simulink model "ik_sim"  (R2019b)
settings: Solver=VariableStepAuto  StartTime=0.0  StopTime=t_k  FixedStep=t_s  MaxStep=t_s  RelTol=1e-3
values from neighbouring files (symbols this model uses):
  d_r = [0.01 0.01 0.01 0.01 0.01 0.01]    [model.mat]
  Fi_b_z = in_rlb(12,1)    [fcn_s_rlb.m]    (also in fcn_s_rub.m = in_rub(12,1); model.mat = [0 2.09439510239 4.18879020479 1.0471975512 3.14159265359 5.)
  l_r = in_rlb(3,1)    [fcn_s_rlb.m]    (also in fcn_s_rub.m = in_rub(3,1); model.mat = [0.36 0.36 0.36 0.36 0.36 0.36])
  O_lb = in_rlb(4:9,1)    [fcn_s_rlb.m]    (also in model.mat = [0 0 0 0 0 0])
  w_lb = in_rlb(11,1)    [fcn_s_rlb.m]    (also in model.mat = 0.195)
  W_lb = 0.205    [model.mat]
  w_ub = in_rub(11,1)    [fcn_s_rub.m]    (also in model.mat = 0.195)
  W_ub = 0.205    [model.mat]
undefined symbols (not defined in the file or in its folder): amp, l_b, om, s_b, t_0, X, Y, Z
libraries: nesl_utility x145, sm_lib x111, dspindex x18
(part 1 of 7)
settings Model: Creator=Vojta  LastModifiedBy=Tom

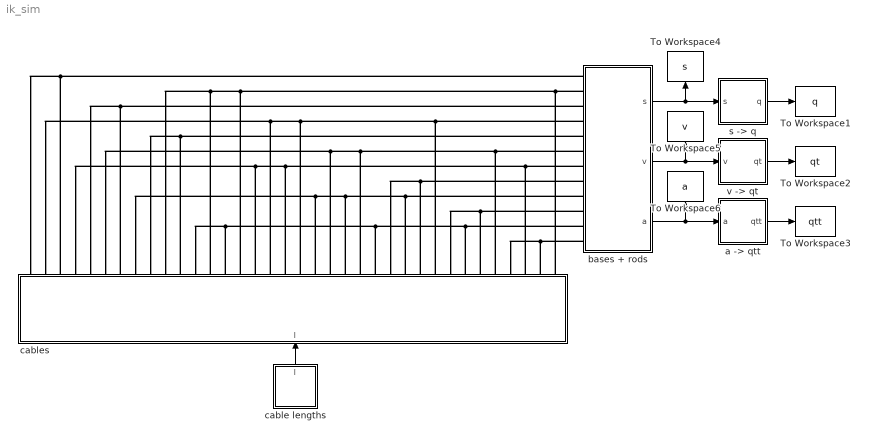
== system ik_sim ==
  To Workspace1 : ToWorkspace  VariableName=q  SampleTime=-1
  To Workspace2 : ToWorkspace  VariableName=qt  SampleTime=-1
  To Workspace3 : ToWorkspace  VariableName=qtt  SampleTime=-1
  To Workspace4 : ToWorkspace  VariableName=s  SampleTime=-1
  To Workspace5 : ToWorkspace  VariableName=v  SampleTime=-1
  To Workspace6 : ToWorkspace  VariableName=a  SampleTime=-1
  "a -> qtt" : MATLAB Function  TreatAsAtomicUnit=on
  bases + rods : Subsystem
  cable lengths : Subsystem
  cables : Subsystem
  "s -> q" : MATLAB Function  TreatAsAtomicUnit=on
  "v -> qt" : MATLAB Function  TreatAsAtomicUnit=on
  wires:
  bases + rods/1(s) -> "s -> q"/1(s), To Workspace4/1
  bases + rods/2(v) -> "v -> qt"/1(v), To Workspace5/1
  bases + rods/3(a) -> "a -> qtt"/1(a), To Workspace6/1
  "a -> qtt"/1(qtt) -> To Workspace3/1
  "v -> qt"/1(qt) -> To Workspace2/1
  "s -> q"/1(q) -> To Workspace1/1
  cable lengths/1(l) -> cables/1(l)
  connections:
  bases + rods/LConn1 -- cables/RConn3 -- cables/RConn1
  bases + rods/LConn2 -- cables/RConn36 -- cables/RConn15 -- cables/RConn10 -- cables/RConn13
  bases + rods/LConn3 -- cables/RConn7 -- cables/RConn5
  bases + rods/LConn4 -- cables/RConn28 -- cables/RConn19 -- cables/RConn17 -- cables/RConn2
  bases + rods/LConn5 -- cables/RConn11 -- cables/RConn9
  bases + rods/LConn6 -- cables/RConn32 -- cables/RConn23 -- cables/RConn21 -- cables/RConn6
  bases + rods/LConn7 -- cables/RConn34 -- cables/RConn18 -- cables/RConn16 -- cables/RConn4
  bases + rods/LConn8 -- cables/RConn27 -- cables/RConn25
  bases + rods/LConn9 -- cables/RConn26 -- cables/RConn22 -- cables/RConn20 -- cables/RConn8
  bases + rods/LConn10 -- cables/RConn31 -- cables/RConn29
  bases + rods/LConn11 -- cables/RConn30 -- cables/RConn24 -- cables/RConn14 -- cables/RConn12
  bases + rods/LConn12 -- cables/RConn35 -- cables/RConn33

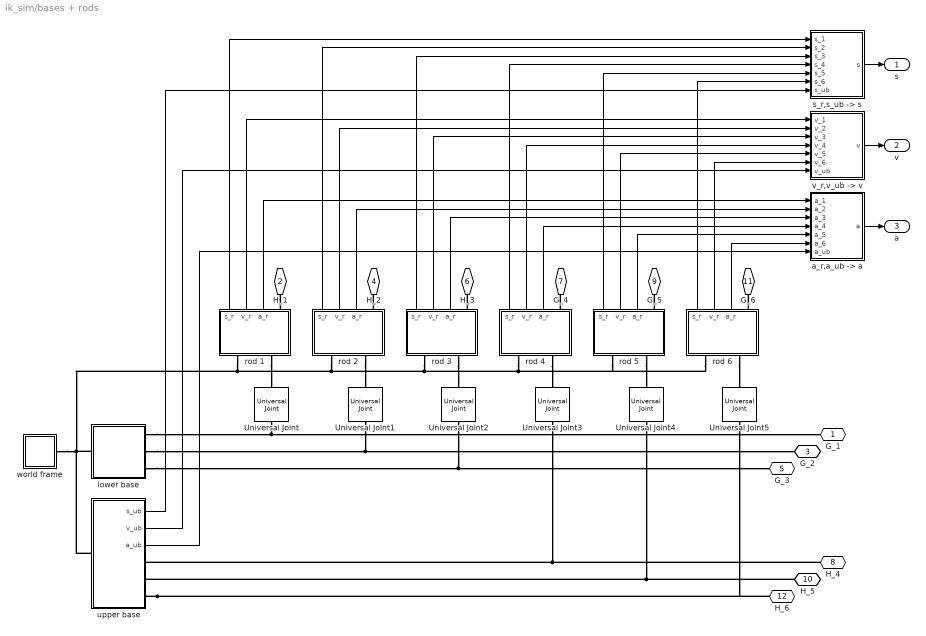
== system ik_sim/bases + rods ==
  Universal Joint{,1..5} (6 alike) : sm_lib/Joints/Universal Joint  JointMode=Normal  SenseConstraintForce=off  SenseConstraintForceX=off  SenseConstraintForceY=off  SenseConstraintForceZ=off  SenseConstraintTorque=off  SenseConstraintTorqueX=off  SenseConstraintTorqueY=off  SenseConstraintTorqueZ=off  SenseTotalForce=off  SenseTotalForceX=off  SenseTotalForceY=off  SenseTotalForceZ=off  SenseTotalTorque=off  SenseTotalTorqueX=off  SenseTotalTorqueY=off  SenseTotalTorqueZ=off  CompositeWrenchDir=FollowerOnBase  CompositeWrenchFrame=BaseFrame  RxEquilibriumPosition=0  RxEquilibriumPositionUnits=deg  RxSpringStiffness=0  RxSpringStiffnessUnits=N*m/deg  RxDampingCoefficient=0  RxDampingCoefficientUnits=N*m/(deg/s)  RxTorqueActuationMode=NoTorque  RxMotionActuationMode=ComputedMotion  RxSensePosition=off  RxSenseVelocity=off  RxSenseAcceleration=off  RxSenseTorqueForce=off  RxSenseLowerLimitTorqueForce=off  RxSenseUpperLimitTorqueForce=off  RxLowerLimitSpecify=off  RxLowerLimitBound=-90  RxLowerLimitBoundUnits=deg  RxLowerLimitStiffness=1e4  RxLowerLimitStiffnessUnits=N*m/deg  RxLowerLimitDamping=10  RxLowerLimitDampingUnits=N*m/(deg/s)  RxLowerLimitTransitionRegionWidth=0.1  RxLowerLimitTransitionRegionWidthUnits=deg  RxUpperLimitSpecify=off  RxUpperLimitBound=90  RxUpperLimitBoundUnits=deg  RxUpperLimitStiffness=1e4  RxUpperLimitStiffnessUnits=N*m/deg  RxUpperLimitDamping=10  RxUpperLimitDampingUnits=N*m/(deg/s)  RxUpperLimitTransitionRegionWidth=0.1  RxUpperLimitTransitionRegionWidthUnits=deg  RxPositionTargetSpecify=off  RxPositionTargetPriority=High  RxPositionTargetValue=0  RxPositionTargetValueUnits=deg  RxVelocityTargetSpecify=off  RxVelocityTargetPriority=High  RxVelocityTargetValue=0  RxVelocityTargetValueUnits=deg/s  RyEquilibriumPosition=0  RyEquilibriumPositionUnits=deg  RySpringStiffness=0  RySpringStiffnessUnits=N*m/deg  RyDampingCoefficient=0  RyDampingCoefficientUnits=N*m/(deg/s)  RyTorqueActuationMode=NoTorque  RyMotionActuationMode=ComputedMotion  RySensePosition=off  RySenseVelocity=off  RySenseAcceleration=off  RySenseTorqueForce=off  RySenseLowerLimitTorqueForce=off  RySenseUpperLimitTorqueForce=off  RyLowerLimitSpecify=off  RyLowerLimitBound=-90  RyLowerLimitBoundUnits=deg  RyLowerLimitStiffness=1e4  RyLowerLimitStiffnessUnits=N*m/deg  RyLowerLimitDamping=10  RyLowerLimitDampingUnits=N*m/(deg/s)  RyLowerLimitTransitionRegionWidth=0.1  RyLowerLimitTransitionRegionWidthUnits=deg  RyUpperLimitSpecify=off  RyUpperLimitBound=90  RyUpperLimitBoundUnits=deg  RyUpperLimitStiffness=1e4  RyUpperLimitStiffnessUnits=N*m/deg  RyUpperLimitDamping=10  RyUpperLimitDampingUnits=N*m/(deg/s)  RyUpperLimitTransitionRegionWidth=0.1  RyUpperLimitTransitionRegionWidthUnits=deg  RyPositionTargetSpecify=off  RyPositionTargetPriority=High  RyPositionTargetValue=0  RyPositionTargetValueUnits=deg  RyVelocityTargetSpecify=off  RyVelocityTargetPriority=High  RyVelocityTargetValue=0  RyVelocityTargetValueUnits=deg/s
      settings: SourceProductName=Simscape Multibody
  "a_r,a_ub -> a" : MATLAB Function  TreatAsAtomicUnit=on
  lower base : Subsystem
  rod 1 : Subsystem  mask{r=1}
  rod 2 : Subsystem  mask{r=2}
  rod 3 : Subsystem  mask{r=3}
  rod 4 : Subsystem  mask{r=4}
  rod 5 : Subsystem  mask{r=5}
  rod 6 : Subsystem  mask{r=6}
  "s_r,s_ub -> s" : MATLAB Function  TreatAsAtomicUnit=on
  upper base : Subsystem
  "v_r,v_ub -> v" : MATLAB Function  TreatAsAtomicUnit=on
  world frame : Subsystem
  G_1 : PMIOPort  Side=Left
  H_1 : PMIOPort  Port=2  Side=Left
  G_2 : PMIOPort  Port=3  Side=Left
  H_2 : PMIOPort  Port=4  Side=Left
  G_3 : PMIOPort  Port=5  Side=Left
  H_3 : PMIOPort  Port=6  Side=Left
  G_4 : PMIOPort  Port=7  Side=Left
  H_4 : PMIOPort  Port=8  Side=Left
  G_5 : PMIOPort  Port=9  Side=Left
  H_5 : PMIOPort  Port=10  Side=Left
  G_6 : PMIOPort  Port=11  Side=Left
  H_6 : PMIOPort  Port=12  Side=Left
  s : Outport
  v : Outport  Port=2
  a : Outport  Port=3
  wires:
  "a_r,a_ub -> a"/1(a) -> a/1
  rod 1/1(s_r) -> "s_r,s_ub -> s"/1(s_1)
  rod 2/1(s_r) -> "s_r,s_ub -> s"/2(s_2)
  rod 3/1(s_r) -> "s_r,s_ub -> s"/3(s_3)
  rod 4/1(s_r) -> "s_r,s_ub -> s"/4(s_4)
  rod 5/1(s_r) -> "s_r,s_ub -> s"/5(s_5)
  rod 6/1(s_r) -> "s_r,s_ub -> s"/6(s_6)
  upper base/1(s_ub) -> "s_r,s_ub -> s"/7(s_ub)
  upper base/2(v_ub) -> "v_r,v_ub -> v"/7(v_ub)
  upper base/3(a_ub) -> "a_r,a_ub -> a"/7(a_ub)
  rod 1/2(v_r) -> "v_r,v_ub -> v"/1(v_1)
  rod 2/2(v_r) -> "v_r,v_ub -> v"/2(v_2)
  rod 3/2(v_r) -> "v_r,v_ub -> v"/3(v_3)
  rod 4/2(v_r) -> "v_r,v_ub -> v"/4(v_4)
  rod 5/2(v_r) -> "v_r,v_ub -> v"/5(v_5)
  rod 6/2(v_r) -> "v_r,v_ub -> v"/6(v_6)
  rod 1/3(a_r) -> "a_r,a_ub -> a"/1(a_1)
  rod 2/3(a_r) -> "a_r,a_ub -> a"/2(a_2)
  rod 3/3(a_r) -> "a_r,a_ub -> a"/3(a_3)
  rod 4/3(a_r) -> "a_r,a_ub -> a"/4(a_4)
  rod 5/3(a_r) -> "a_r,a_ub -> a"/5(a_5)
  rod 6/3(a_r) -> "a_r,a_ub -> a"/6(a_6)
  "v_r,v_ub -> v"/1(v) -> v/1
  "s_r,s_ub -> s"/1(s) -> s/1
  connections:
  Universal Joint2/LConn1 -- G_3/RConn1 -- lower base/RConn3
  Universal Joint1/LConn1 -- G_2/RConn1 -- lower base/RConn2
  H_4/RConn1 -- Universal Joint3/LConn1 -- upper base/RConn1
  Universal Joint/LConn1 -- G_1/RConn1 -- lower base/RConn1
  rod 1/LConn1 -- rod 2/LConn1 -- rod 3/LConn1 -- rod 4/LConn1 -- rod 6/LConn1 -- rod 5/LConn1 -- world frame/RConn1 -- upper base/LConn1 -- lower base/LConn1
  upper base/RConn3 -- H_6/RConn1 -- Universal Joint5/LConn1
  H_5/RConn1 -- Universal Joint4/LConn1 -- upper base/RConn2
  rod 1/RConn1 -- H_1/RConn1
  rod 1/LConn2 -- Universal Joint/RConn1
  rod 2/LConn2 -- Universal Joint1/RConn1
  rod 3/LConn2 -- Universal Joint2/RConn1
  rod 2/RConn1 -- H_2/RConn1
  rod 3/RConn1 -- H_3/RConn1
  rod 4/LConn2 -- Universal Joint3/RConn1
  rod 4/RConn1 -- G_4/RConn1
  rod 5/LConn2 -- Universal Joint4/RConn1
  rod 6/LConn2 -- Universal Joint5/RConn1
  rod 5/RConn1 -- G_5/RConn1
  rod 6/RConn1 -- G_6/RConn1

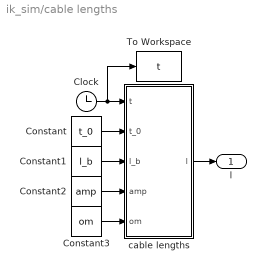
== system ik_sim/cable lengths ==
  Clock : Clock
  Constant : Constant  Value=t_0
  Constant1 : Constant  Value=l_b
  Constant2 : Constant  Value=amp
  Constant3 : Constant  Value=om
  To Workspace : ToWorkspace  VariableName=t  SampleTime=-1
  cable lengths : MATLAB Function  TreatAsAtomicUnit=on
  l : Outport
  wires:
  Constant/1 -> cable lengths/2(t_0)
  Constant1/1 -> cable lengths/3(l_b)
  Constant2/1 -> cable lengths/4(amp)
  Constant3/1 -> cable lengths/5(om)
  Clock/1 -> To Workspace/1, cable lengths/1(t)
  cable lengths/1(l) -> l/1

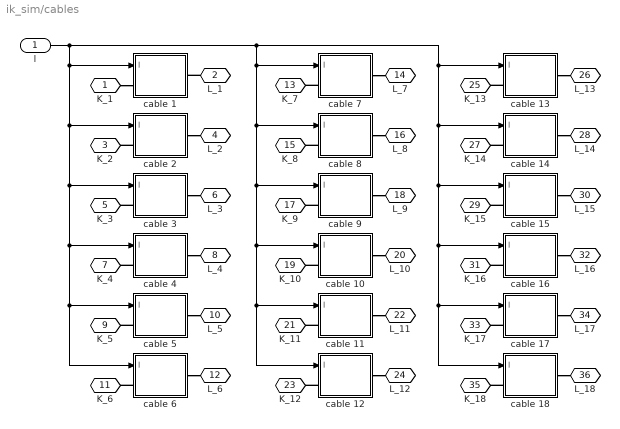
== system ik_sim/cables ==
  l : Inport
  cable 1 : Subsystem  mask{c=1}
  cable 10 : Subsystem  mask{c=10}
  cable 11 : Subsystem  mask{c=11}
  cable 12 : Subsystem  mask{c=12}
  cable 13 : Subsystem  mask{c=13}
  cable 14 : Subsystem  mask{c=14}
  cable 15 : Subsystem  mask{c=15}
  cable 16 : Subsystem  mask{c=16}
  cable 17 : Subsystem  mask{c=17}
  cable 18 : Subsystem  mask{c=18}
  cable 2 : Subsystem  mask{c=2}
  cable 3 : Subsystem  mask{c=3}
  cable 4 : Subsystem  mask{c=4}
  cable 5 : Subsystem  mask{c=5}
  cable 6 : Subsystem  mask{c=6}
  cable 7 : Subsystem  mask{c=7}
  cable 8 : Subsystem  mask{c=8}
  cable 9 : Subsystem  mask{c=9}
  K_1 : PMIOPort  Side=Right
  L_1 : PMIOPort  Port=2  Side=Right
  K_2 : PMIOPort  Port=3  Side=Right
  L_2 : PMIOPort  Port=4  Side=Right
  K_3 : PMIOPort  Port=5  Side=Right
  L_3 : PMIOPort  Port=6  Side=Right
  K_4 : PMIOPort  Port=7  Side=Right
  L_4 : PMIOPort  Port=8  Side=Right
  K_5 : PMIOPort  Port=9  Side=Right
  L_5 : PMIOPort  Port=10  Side=Right
  K_6 : PMIOPort  Port=11  Side=Right
  L_6 : PMIOPort  Port=12  Side=Right
  K_7 : PMIOPort  Port=13  Side=Right
  L_7 : PMIOPort  Port=14  Side=Right
  K_8 : PMIOPort  Port=15  Side=Right
  L_8 : PMIOPort  Port=16  Side=Right
  K_9 : PMIOPort  Port=17  Side=Right
  L_9 : PMIOPort  Port=18  Side=Right
  K_10 : PMIOPort  Port=19  Side=Right
  L_10 : PMIOPort  Port=20  Side=Right
  K_11 : PMIOPort  Port=21  Side=Right
  L_11 : PMIOPort  Port=22  Side=Right
  K_12 : PMIOPort  Port=23  Side=Right
  L_12 : PMIOPort  Port=24  Side=Right
  K_13 : PMIOPort  Port=25  Side=Right
  L_13 : PMIOPort  Port=26  Side=Right
  K_14 : PMIOPort  Port=27  Side=Right
  L_14 : PMIOPort  Port=28  Side=Right
  K_15 : PMIOPort  Port=29  Side=Right
  L_15 : PMIOPort  Port=30  Side=Right
  K_16 : PMIOPort  Port=31  Side=Right
  L_16 : PMIOPort  Port=32  Side=Right
  K_17 : PMIOPort  Port=33  Side=Right
  L_17 : PMIOPort  Port=34  Side=Right
  K_18 : PMIOPort  Port=35  Side=Right
  L_18 : PMIOPort  Port=36  Side=Right
  wires:
  l/1 -> cable 1/1(l), cable 2/1(l), cable 3/1(l), cable 4/1(l), cable 5/1(l), cable 6/1(l), cable 7/1(l), cable 8/1(l), cable 9/1(l), cable 10/1(l), cable 12/1(l), cable 11/1(l), cable 13/1(l), cable 14/1(l), cable 15/1(l), cable 16/1(l), cable 18/1(l), cable 17/1(l)
  connections:
  L_1/RConn1 -- cable 1/RConn1
  K_1/RConn1 -- cable 1/LConn1
  cable 2/LConn1 -- K_2/RConn1
  cable 2/RConn1 -- L_2/RConn1
  cable 3/LConn1 -- K_3/RConn1
  cable 4/LConn1 -- K_4/RConn1
  cable 5/LConn1 -- K_5/RConn1
  cable 6/LConn1 -- K_6/RConn1
  cable 9/RConn1 -- L_9/RConn1
  cable 9/LConn1 -- K_9/RConn1
  cable 7/RConn1 -- L_7/RConn1
  cable 7/LConn1 -- K_7/RConn1
  cable 8/RConn1 -- L_8/RConn1
  cable 8/LConn1 -- K_8/RConn1
  cable 11/LConn1 -- K_11/RConn1
  cable 10/RConn1 -- L_10/RConn1
  cable 11/RConn1 -- L_11/RConn1
  cable 12/RConn1 -- L_12/RConn1
  cable 12/LConn1 -- K_12/RConn1
  cable 10/LConn1 -- K_10/RConn1
  cable 13/LConn1 -- K_13/RConn1
  cable 14/RConn1 -- L_14/RConn1
  cable 13/RConn1 -- L_13/RConn1
  cable 15/RConn1 -- L_15/RConn1
  cable 14/LConn1 -- K_14/RConn1
  cable 15/LConn1 -- K_15/RConn1
  cable 17/RConn1 -- L_17/RConn1
  cable 18/LConn1 -- K_18/RConn1
  cable 16/RConn1 -- L_16/RConn1
  cable 17/LConn1 -- K_17/RConn1
  cable 18/RConn1 -- L_18/RConn1
  cable 16/LConn1 -- K_16/RConn1
  cable 3/RConn1 -- L_3/RConn1
  cable 4/RConn1 -- L_4/RConn1
  cable 5/RConn1 -- L_5/RConn1
  cable 6/RConn1 -- L_6/RConn1

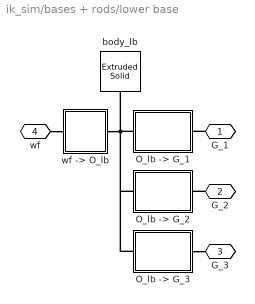
== system ik_sim/bases + rods/lower base ==
  "O_lb -> G_1" : Subsystem
  "O_lb -> G_2" : Subsystem
  "O_lb -> G_3" : Subsystem
  body_lb : sm_lib/Body Elements/Extruded Solid  GraphicAmbientColor=[0.15 0.15 0.15 1.0]  BasedOnType=Density  CenterOfMass=[0 0 0]  CenterOfMassUnits=m  GraphicDiffuseColor=[0.5,0.5,0.5]  ExtrusionCrossSection=[1 1; -1 1; -1 -1; 1 -1]  ExtrusionCrossSectionUnits=m  Density=Ro_lb  DensityUnits=kg/m^3  DoExposeReferenceFrame=on  GraphicEmissiveColor=[0.0 0.0 0.0 1.0]  ExportEntireGeometry=off  ExtrusionLength=t_lb  ExtrusionLengthUnits=m  ExtrusionType=Regular  SerializedFrames=<Frames/>  MarkerShape=Sphere  MarkerSize=10  GraphicType=FromGeometry  InertiaType=CalculateFromGeometry  Mass=1  MassUnits=kg  MomentsOfInertia=[1 1 1]  MomentsOfInertiaUnits=kg*m^2  PolygonNumSides=6  GraphicOpacity=1  PolygonOuterRadius=(W_lb/2)/cosd(30)  PolygonOuterRadiusUnits=m  ProductsOfInertia=[0 0 0]  ProductsOfInertiaUnits=kg*m^2  GraphicShininess=75  GraphicSpecularColor=[0.5 0.5 0.5 1.0]  GraphicVisPropType=SimpleVisualProperties
      settings: SourceProductName=Simscape Multibody
  "wf -> O_lb" : Subsystem
  G_1 : PMIOPort  Side=Right
  G_2 : PMIOPort  Port=2  Side=Right
  G_3 : PMIOPort  Port=3  Side=Right
  wf : PMIOPort  Port=4  Side=Left
  connections:
  wf/RConn1 -- "wf -> O_lb"/LConn1
  "wf -> O_lb"/RConn1 -- "O_lb -> G_3"/LConn1 -- "O_lb -> G_2"/LConn1 -- body_lb/RConn1 -- "O_lb -> G_1"/LConn1
  G_1/RConn1 -- "O_lb -> G_1"/RConn1
  G_2/RConn1 -- "O_lb -> G_2"/RConn1
  "O_lb -> G_3"/RConn1 -- G_3/RConn1

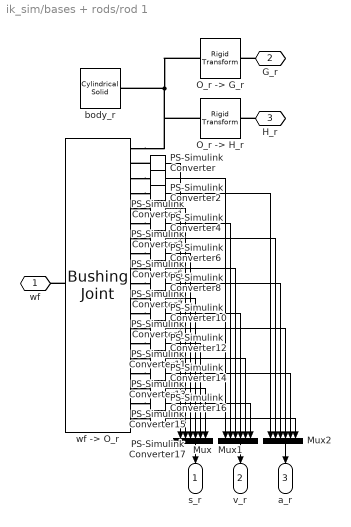
== system ik_sim/bases + rods/rod 1 ==
  Mux : Mux  Inputs=6
  Mux1 : Mux  Inputs=6
  Mux2 : Mux  Inputs=6
  "O_r -> G_r" : sm_lib/Frames and Transforms/Rigid Transform  TranslationMethod=StandardAxis  TranslationStandardOffset=l_r(r)/2  TranslationLengthUnit=m  TranslationStandardAxis=-Z  TranslationCartesianOffset=[0 0 0]  TranslationROffset=0  TranslationROffsetUnits=m  TranslationZOffset=0  TranslationZOffsetUnits=m  TranslationThetaOffset=0  TranslationThetaOffsetUnits=deg  RotationMethod=None  RotationAngleUnits=deg  RotationStandardAxis=+Z  RotationAngle=0.0  RotationArbitraryAxis=[0 0 1]  FollAlignAxisA=+X  BaseAlignAxisA=+Y  FollAlignAxisB=+Y  BaseAlignAxisB=+Z  RotationSequenceAxes=FollowerAxes  RotationSequence=XYX  RotationSequenceAngles=[0 0 0]  RotationSequenceAnglesUnits=deg  RotationMatrix=[1 0 0; 0 1 0; 0 0 1]
  "O_r -> H_r" : sm_lib/Frames and Transforms/Rigid Transform  TranslationMethod=StandardAxis  TranslationStandardOffset=l_r(r)/2  TranslationLengthUnit=m  TranslationStandardAxis=+Z  TranslationCartesianOffset=[0 0 0]  TranslationROffset=0  TranslationROffsetUnits=m  TranslationZOffset=0  TranslationZOffsetUnits=m  TranslationThetaOffset=0  TranslationThetaOffsetUnits=deg  RotationMethod=None  RotationAngleUnits=deg  RotationStandardAxis=+Z  RotationAngle=0.0  RotationArbitraryAxis=[0 0 1]  FollAlignAxisA=+X  BaseAlignAxisA=+Y  FollAlignAxisB=+Y  BaseAlignAxisB=+Z  RotationSequenceAxes=FollowerAxes  RotationSequence=XYX  RotationSequenceAngles=[0 0 0]  RotationSequenceAnglesUnits=deg  RotationMatrix=[1 0 0; 0 1 0; 0 0 1]
  PS-Simulink Converter{,1..17} (18 alike) : nesl_utility/PS-Simulink Converter  PhysicalDomain=network_engine_domain  SubClassName=ps_output  LeftPortType=input  RightPortType=output  PseudoPeriodic=off  Frequencies=[]  Unit=inherit  AffineConversion=off
  body_r : sm_lib/Body Elements/Cylindrical Solid  GraphicAmbientColor=[0.15 0.15 0.15 1.0]  BasedOnType=Density  CenterOfMass=[0 0 0]  CenterOfMassUnits=m  GraphicDiffuseColor=[0.5,0.5,0.5]  CylinderLength=l_r(r)  CylinderLengthUnits=m  CylinderRadius=d_r(r)/2  CylinderRadiusUnits=m  Density=Ro_r  DensityUnits=kg/m^3  DoExposeReferenceFrame=on  GraphicEmissiveColor=[0.0 0.0 0.0 1.0]  ExportEntireGeometry=off  SerializedFrames=<Frames/>  MarkerShape=Sphere  MarkerSize=10  GraphicType=FromGeometry  InertiaType=CalculateFromGeometry  Mass=1  MassUnits=kg  MomentsOfInertia=[1 1 1]  MomentsOfInertiaUnits=kg*m^2  GraphicOpacity=1  ProductsOfInertia=[0 0 0]  ProductsOfInertiaUnits=kg*m^2  GraphicShininess=75  GraphicSpecularColor=[0.5 0.5 0.5 1.0]  GraphicVisPropType=SimpleVisualProperties
  "wf -> O_r" : sm_lib/Joints/Bushing Joint  JointMode=Normal  SenseConstraintForce=off  SenseConstraintForceX=off  SenseConstraintForceY=off  SenseConstraintForceZ=off  SenseConstraintTorque=off  SenseConstraintTorqueX=off  SenseConstraintTorqueY=off  SenseConstraintTorqueZ=off  SenseTotalForce=off  SenseTotalForceX=off  SenseTotalForceY=off  SenseTotalForceZ=off  SenseTotalTorque=off  SenseTotalTorqueX=off  SenseTotalTorqueY=off  SenseTotalTorqueZ=off  CompositeWrenchDir=FollowerOnBase  CompositeWrenchFrame=BaseFrame  PxEquilibriumPosition=0  PxEquilibriumPositionUnits=m  PxSpringStiffness=0  PxSpringStiffnessUnits=N/m  PxDampingCoefficient=0  PxDampingCoefficientUnits=N/(m/s)  PxTorqueActuationMode=NoTorque  PxMotionActuationMode=ComputedMotion  PxSensePosition=on  PxSenseVelocity=on  PxSenseAcceleration=on  PxSenseTorqueForce=off  PxSenseLowerLimitTorqueForce=off  PxSenseUpperLimitTorqueForce=off  PxLowerLimitSpecify=off  PxLowerLimitBound=-1  PxLowerLimitBoundUnits=m  PxLowerLimitStiffness=1e6  PxLowerLimitStiffnessUnits=N/m  PxLowerLimitDamping=1e3  PxLowerLimitDampingUnits=N/(m/s)  PxLowerLimitTransitionRegionWidth=1e-4  PxLowerLimitTransitionRegionWidthUnits=m  PxUpperLimitSpecify=off  PxUpperLimitBound=1  PxUpperLimitBoundUnits=m  PxUpperLimitStiffness=1e6  PxUpperLimitStiffnessUnits=N/m  PxUpperLimitDamping=1e3  PxUpperLimitDampingUnits=N/(m/s)  PxUpperLimitTransitionRegionWidth=1e-4  PxUpperLimitTransitionRegionWidthUnits=m  PxPositionTargetSpecify=on  PxPositionTargetPriority=Low  PxPositionTargetValue=s_b(1,r)  PxPositionTargetValueUnits=m  PxVelocityTargetSpecify=off  PxVelocityTargetPriority=High  PxVelocityTargetValue=0  PxVelocityTargetValueUnits=m/s  PyEquilibriumPosition=0  PyEquilibriumPositionUnits=m  PySpringStiffness=0  PySpringStiffnessUnits=N/m  PyDampingCoefficient=0  PyDampingCoefficientUnits=N/(m/s)  PyTorqueActuationMode=NoTorque  PyMotionActuationMode=ComputedMotion  PySensePosition=on  PySenseVelocity=on  PySenseAcceleration=on  PySenseTorqueForce=off  PySenseLowerLimitTorqueForce=off  PySenseUpperLimitTorqueForce=off  PyLowerLimitSpecify=off  PyLowerLimitBound=-1  PyLowerLimitBoundUnits=m  PyLowerLimitStiffness=1e6  PyLowerLimitStiffnessUnits=N/m  PyLowerLimitDamping=1e3  PyLowerLimitDampingUnits=N/(m/s)  PyLowerLimitTransitionRegionWidth=1e-4  PyLowerLimitTransitionRegionWidthUnits=m  PyUpperLimitSpecify=off  PyUpperLimitBound=1  PyUpperLimitBoundUnits=m  PyUpperLimitStiffness=1e6  PyUpperLimitStiffnessUnits=N/m  PyUpperLimitDamping=1e3  PyUpperLimitDampingUnits=N/(m/s)  PyUpperLimitTransitionRegionWidth=1e-4  PyUpperLimitTransitionRegionWidthUnits=m  PyPositionTargetSpecify=on  PyPositionTargetPriority=Low  PyPositionTargetValue=s_b(2,r)  PyPositionTargetValueUnits=m  PyVelocityTargetSpecify=off  PyVelocityTargetPriority=High  PyVelocityTargetValue=0  PyVelocityTargetValueUnits=m/s  PzEquilibriumPosition=0  PzEquilibriumPositionUnits=m  PzSpringStiffness=0  PzSpringStiffnessUnits=N/m  PzDampingCoefficient=0  PzDampingCoefficientUnits=N/(m/s)  PzTorqueActuationMode=NoTorque  PzMotionActuationMode=ComputedMotion  PzSensePosition=on  PzSenseVelocity=on  PzSenseAcceleration=on  PzSenseTorqueForce=off  PzSenseLowerLimitTorqueForce=off  PzSenseUpperLimitTorqueForce=off  PzLowerLimitSpecify=off  PzLowerLimitBound=-1  PzLowerLimitBoundUnits=m  PzLowerLimitStiffness=1e6  PzLowerLimitStiffnessUnits=N/m  PzLowerLimitDamping=1e3  PzLowerLimitDampingUnits=N/(m/s)  PzLowerLimitTransitionRegionWidth=1e-4  PzLowerLimitTransitionRegionWidthUnits=m  PzUpperLimitSpecify=off  PzUpperLimitBound=1  PzUpperLimitBoundUnits=m  PzUpperLimitStiffness=1e6  PzUpperLimitStiffnessUnits=N/m  PzUpperLimitDamping=1e3  PzUpperLimitDampingUnits=N/(m/s)  PzUpperLimitTransitionRegionWidth=1e-4  PzUpperLimitTransitionRegionWidthUnits=m  PzPositionTargetSpecify=on  PzPositionTargetPriority=Low  PzPositionTargetValue=s_b(3,r)  PzPositionTargetValueUnits=m  PzVelocityTargetSpecify=off  PzVelocityTargetPriority=High  PzVelocityTargetValue=0  PzVelocityTargetValueUnits=m/s  RxEquilibriumPosition=0  RxEquilibriumPositionUnits=deg  RxSpringStiffness=0  RxSpringStiffnessUnits=N*m/deg  RxDampingCoefficient=0  RxDampingCoefficientUnits=N*m/(deg/s)  RxTorqueActuationMode=NoTorque  RxMotionActuationMode=ComputedMotion  RxSensePosition=on  RxSenseVelocity=on  RxSenseAcceleration=on  RxSenseTorqueForce=off  RxSenseLowerLimitTorqueForce=off  RxSenseUpperLimitTorqueForce=off  RxLowerLimitSpecify=off  RxLowerLimitBound=-90  RxLowerLimitBoundUnits=deg  RxLowerLimitStiffness=1e4  RxLowerLimitStiffnessUnits=N*m/deg  RxLowerLimitDamping=10  RxLowerLimitDampingUnits=N*m/(deg/s)  RxLowerLimitTransitionRegionWidth=0.1  RxLowerLimitTransitionRegionWidthUnits=deg  RxUpperLimitSpecify=off  RxUpperLimitBound=90  RxUpperLimitBoundUnits=deg  RxUpperLimitStiffness=1e4  RxUpperLimitStiffnessUnits=N*m/deg  RxUpperLimitDamping=10  RxUpperLimitDampingUnits=N*m/(deg/s)  RxUpperLimitTransitionRegionWidth=0.1  RxUpperLimitTransitionRegionWidthUnits=deg  RxPositionTargetSpecify=on  RxPositionTargetPriority=Low  RxPositionTargetValue=s_b(4,r)  RxPositionTargetValueUnits=rad  RxVelocityTargetSpecify=off  RxVelocityTargetPriority=High  RxVelocityTargetValue=0  RxVelocityTargetValueUnits=rad/s  RyEquilibriumPosition=0  RyEquilibriumPositionUnits=deg  RySpringStiffness=0  RySpringStiffnessUnits=N*m/deg  RyDampingCoefficient=0  RyDampingCoefficientUnits=N*m/(deg/s)  RyTorqueActuationMode=NoTorque  RyMotionActuationMode=ComputedMotion  RySensePosition=on  RySenseVelocity=on  RySenseAcceleration=on  RySenseTorqueForce=off  RySenseLowerLimitTorqueForce=off  RySenseUpperLimitTorqueForce=off  RyLowerLimitSpecify=off  RyLowerLimitBound=-90  RyLowerLimitBoundUnits=deg  RyLowerLimitStiffness=1e4  RyLowerLimitStiffnessUnits=N*m/deg  RyLowerLimitDamping=10  RyLowerLimitDampingUnits=N*m/(deg/s)  RyLowerLimitTransitionRegionWidth=0.1  RyLowerLimitTransitionRegionWidthUnits=deg  RyUpperLimitSpecify=off  RyUpperLimitBound=90  RyUpperLimitBoundUnits=deg  RyUpperLimitStiffness=1e4  RyUpperLimitStiffnessUnits=N*m/deg  RyUpperLimitDamping=10  RyUpperLimitDampingUnits=N*m/(deg/s)  RyUpperLimitTransitionRegionWidth=0.1  RyUpperLimitTransitionRegionWidthUnits=deg  RyPositionTargetSpecify=on  RyPositionTargetPriority=Low  RyPositionTargetValue=s_b(5,r)  RyPositionTargetValueUnits=rad  RyVelocityTargetSpecify=off  RyVelocityTargetPriority=High  RyVelocityTargetValue=0  RyVelocityTargetValueUnits=rad/s  RzEquilibriumPosition=0  RzEquilibriumPositionUnits=deg  RzSpringStiffness=0  RzSpringStiffnessUnits=N*m/deg  RzDampingCoefficient=0  RzDampingCoefficientUnits=N*m/(deg/s)  RzTorqueActuationMode=NoTorque  RzMotionActuationMode=ComputedMotion  RzSensePosition=on  RzSenseVelocity=on  RzSenseAcceleration=on  RzSenseTorqueForce=off  RzSenseLowerLimitTorqueForce=off  RzSenseUpperLimitTorqueForce=off  RzLowerLimitSpecify=off  RzLowerLimitBound=-90  RzLowerLimitBoundUnits=deg  RzLowerLimitStiffness=1e4  RzLowerLimitStiffnessUnits=N*m/deg  RzLowerLimitDamping=10  RzLowerLimitDampingUnits=N*m/(deg/s)  RzLowerLimitTransitionRegionWidth=0.1  RzLowerLimitTransitionRegionWidthUnits=deg  RzUpperLimitSpecify=off  RzUpperLimitBound=90  RzUpperLimitBoundUnits=deg  RzUpperLimitStiffness=1e4  RzUpperLimitStiffnessUnits=N*m/deg  RzUpperLimitDamping=10  RzUpperLimitDampingUnits=N*m/(deg/s)  RzUpperLimitTransitionRegionWidth=0.1  RzUpperLimitTransitionRegionWidthUnits=deg  RzPositionTargetSpecify=on  RzPositionTargetPriority=Low  RzPositionTargetValue=s_b(6,r)  RzPositionTargetValueUnits=rad  RzVelocityTargetSpecify=off  RzVelocityTargetPriority=High  RzVelocityTargetValue=0  RzVelocityTargetValueUnits=rad/s
      settings: SourceProductName=Simscape Multibody
  wf : PMIOPort  Side=Left
  G_r : PMIOPort  Port=2  Side=Left
  H_r : PMIOPort  Port=3  Side=Right
  s_r : Outport
  v_r : Outport  Port=2
  a_r : Outport  Port=3
  wires:
  PS-Simulink Converter/1 -> Mux/1
  PS-Simulink Converter3/1 -> Mux/2
  PS-Simulink Converter6/1 -> Mux/3
  PS-Simulink Converter9/1 -> Mux/4
  PS-Simulink Converter12/1 -> Mux/5
  PS-Simulink Converter15/1 -> Mux/6
  Mux/1 -> s_r/1
  PS-Simulink Converter1/1 -> Mux1/1
  PS-Simulink Converter4/1 -> Mux1/2
  PS-Simulink Converter7/1 -> Mux1/3
  PS-Simulink Converter10/1 -> Mux1/4
  PS-Simulink Converter13/1 -> Mux1/5
  PS-Simulink Converter16/1 -> Mux1/6
  Mux1/1 -> v_r/1
  PS-Simulink Converter2/1 -> Mux2/1
  PS-Simulink Converter5/1 -> Mux2/2
  PS-Simulink Converter8/1 -> Mux2/3
  PS-Simulink Converter11/1 -> Mux2/4
  PS-Simulink Converter14/1 -> Mux2/5
  PS-Simulink Converter17/1 -> Mux2/6
  Mux2/1 -> a_r/1
  connections:
  "wf -> O_r"/LConn1 -- wf/RConn1
  "O_r -> G_r"/LConn1 -- "wf -> O_r"/RConn1 -- "O_r -> H_r"/LConn1 -- body_r/RConn1
  H_r/RConn1 -- "O_r -> H_r"/RConn1
  G_r/RConn1 -- "O_r -> G_r"/RConn1
  PS-Simulink Converter/LConn1 -- "wf -> O_r"/RConn2
  "wf -> O_r"/RConn3 -- PS-Simulink Converter1/LConn1
  "wf -> O_r"/RConn4 -- PS-Simulink Converter2/LConn1
  "wf -> O_r"/RConn5 -- PS-Simulink Converter3/LConn1
  "wf -> O_r"/RConn6 -- PS-Simulink Converter4/LConn1
  "wf -> O_r"/RConn7 -- PS-Simulink Converter5/LConn1
  "wf -> O_r"/RConn8 -- PS-Simulink Converter6/LConn1
  "wf -> O_r"/RConn9 -- PS-Simulink Converter7/LConn1
  "wf -> O_r"/RConn10 -- PS-Simulink Converter8/LConn1
  "wf -> O_r"/RConn11 -- PS-Simulink Converter9/LConn1
  "wf -> O_r"/RConn12 -- PS-Simulink Converter10/LConn1
  "wf -> O_r"/RConn13 -- PS-Simulink Converter11/LConn1
  "wf -> O_r"/RConn14 -- PS-Simulink Converter12/LConn1
  "wf -> O_r"/RConn15 -- PS-Simulink Converter13/LConn1
  "wf -> O_r"/RConn16 -- PS-Simulink Converter14/LConn1
  "wf -> O_r"/RConn17 -- PS-Simulink Converter15/LConn1
  "wf -> O_r"/RConn18 -- PS-Simulink Converter16/LConn1
  "wf -> O_r"/RConn19 -- PS-Simulink Converter17/LConn1

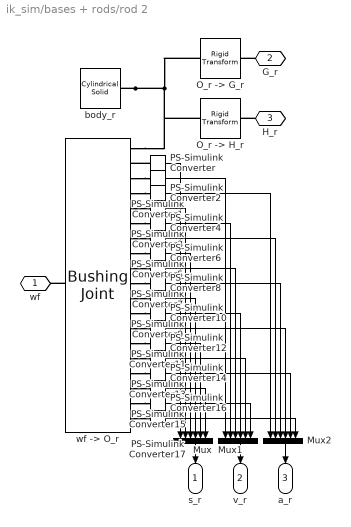
== system ik_sim/bases + rods/rod 2 ==
  Mux : Mux  Inputs=6
  Mux1 : Mux  Inputs=6
  Mux2 : Mux  Inputs=6
  "O_r -> G_r" : sm_lib/Frames and Transforms/Rigid Transform  TranslationMethod=StandardAxis  TranslationStandardOffset=l_r(r)/2  TranslationLengthUnit=m  TranslationStandardAxis=-Z  TranslationCartesianOffset=[0 0 0]  TranslationROffset=0  TranslationROffsetUnits=m  TranslationZOffset=0  TranslationZOffsetUnits=m  TranslationThetaOffset=0  TranslationThetaOffsetUnits=deg  RotationMethod=None  RotationAngleUnits=deg  RotationStandardAxis=+Z  RotationAngle=0.0  RotationArbitraryAxis=[0 0 1]  FollAlignAxisA=+X  BaseAlignAxisA=+Y  FollAlignAxisB=+Y  BaseAlignAxisB=+Z  RotationSequenceAxes=FollowerAxes  RotationSequence=XYX  RotationSequenceAngles=[0 0 0]  RotationSequenceAnglesUnits=deg  RotationMatrix=[1 0 0; 0 1 0; 0 0 1]
  "O_r -> H_r" : sm_lib/Frames and Transforms/Rigid Transform  TranslationMethod=StandardAxis  TranslationStandardOffset=l_r(r)/2  TranslationLengthUnit=m  TranslationStandardAxis=+Z  TranslationCartesianOffset=[0 0 0]  TranslationROffset=0  TranslationROffsetUnits=m  TranslationZOffset=0  TranslationZOffsetUnits=m  TranslationThetaOffset=0  TranslationThetaOffsetUnits=deg  RotationMethod=None  RotationAngleUnits=deg  RotationStandardAxis=+Z  RotationAngle=0.0  RotationArbitraryAxis=[0 0 1]  FollAlignAxisA=+X  BaseAlignAxisA=+Y  FollAlignAxisB=+Y  BaseAlignAxisB=+Z  RotationSequenceAxes=FollowerAxes  RotationSequence=XYX  RotationSequenceAngles=[0 0 0]  RotationSequenceAnglesUnits=deg  RotationMatrix=[1 0 0; 0 1 0; 0 0 1]
  PS-Simulink Converter{,1..17} (18 alike) : nesl_utility/PS-Simulink Converter  PhysicalDomain=network_engine_domain  SubClassName=ps_output  LeftPortType=input  RightPortType=output  PseudoPeriodic=off  Frequencies=[]  Unit=inherit  AffineConversion=off
  body_r : sm_lib/Body Elements/Cylindrical Solid  GraphicAmbientColor=[0.15 0.15 0.15 1.0]  BasedOnType=Density  CenterOfMass=[0 0 0]  CenterOfMassUnits=m  GraphicDiffuseColor=[0.5,0.5,0.5]  CylinderLength=l_r(r)  CylinderLengthUnits=m  CylinderRadius=d_r(r)/2  CylinderRadiusUnits=m  Density=Ro_r  DensityUnits=kg/m^3  DoExposeReferenceFrame=on  GraphicEmissiveColor=[0.0 0.0 0.0 1.0]  ExportEntireGeometry=off  SerializedFrames=<Frames/>  MarkerShape=Sphere  MarkerSize=10  GraphicType=FromGeometry  InertiaType=CalculateFromGeometry  Mass=1  MassUnits=kg  MomentsOfInertia=[1 1 1]  MomentsOfInertiaUnits=kg*m^2  GraphicOpacity=1  ProductsOfInertia=[0 0 0]  ProductsOfInertiaUnits=kg*m^2  GraphicShininess=75  GraphicSpecularColor=[0.5 0.5 0.5 1.0]  GraphicVisPropType=SimpleVisualProperties
  "wf -> O_r" : sm_lib/Joints/Bushing Joint  JointMode=Normal  SenseConstraintForce=off  SenseConstraintForceX=off  SenseConstraintForceY=off  SenseConstraintForceZ=off  SenseConstraintTorque=off  SenseConstraintTorqueX=off  SenseConstraintTorqueY=off  SenseConstraintTorqueZ=off  SenseTotalForce=off  SenseTotalForceX=off  SenseTotalForceY=off  SenseTotalForceZ=off  SenseTotalTorque=off  SenseTotalTorqueX=off  SenseTotalTorqueY=off  SenseTotalTorqueZ=off  CompositeWrenchDir=FollowerOnBase  CompositeWrenchFrame=BaseFrame  PxEquilibriumPosition=0  PxEquilibriumPositionUnits=m  PxSpringStiffness=0  PxSpringStiffnessUnits=N/m  PxDampingCoefficient=0  PxDampingCoefficientUnits=N/(m/s)  PxTorqueActuationMode=NoTorque  PxMotionActuationMode=ComputedMotion  PxSensePosition=on  PxSenseVelocity=on  PxSenseAcceleration=on  PxSenseTorqueForce=off  PxSenseLowerLimitTorqueForce=off  PxSenseUpperLimitTorqueForce=off  PxLowerLimitSpecify=off  PxLowerLimitBound=-1  PxLowerLimitBoundUnits=m  PxLowerLimitStiffness=1e6  PxLowerLimitStiffnessUnits=N/m  PxLowerLimitDamping=1e3  PxLowerLimitDampingUnits=N/(m/s)  PxLowerLimitTransitionRegionWidth=1e-4  PxLowerLimitTransitionRegionWidthUnits=m  PxUpperLimitSpecify=off  PxUpperLimitBound=1  PxUpperLimitBoundUnits=m  PxUpperLimitStiffness=1e6  PxUpperLimitStiffnessUnits=N/m  PxUpperLimitDamping=1e3  PxUpperLimitDampingUnits=N/(m/s)  PxUpperLimitTransitionRegionWidth=1e-4  PxUpperLimitTransitionRegionWidthUnits=m  PxPositionTargetSpecify=on  PxPositionTargetPriority=Low  PxPositionTargetValue=s_b(1,r)  PxPositionTargetValueUnits=m  PxVelocityTargetSpecify=off  PxVelocityTargetPriority=High  PxVelocityTargetValue=0  PxVelocityTargetValueUnits=m/s  PyEquilibriumPosition=0  PyEquilibriumPositionUnits=m  PySpringStiffness=0  PySpringStiffnessUnits=N/m  PyDampingCoefficient=0  PyDampingCoefficientUnits=N/(m/s)  PyTorqueActuationMode=NoTorque  PyMotionActuationMode=ComputedMotion  PySensePosition=on  PySenseVelocity=on  PySenseAcceleration=on  PySenseTorqueForce=off  PySenseLowerLimitTorqueForce=off  PySenseUpperLimitTorqueForce=off  PyLowerLimitSpecify=off  PyLowerLimitBound=-1  PyLowerLimitBoundUnits=m  PyLowerLimitStiffness=1e6  PyLowerLimitStiffnessUnits=N/m  PyLowerLimitDamping=1e3  PyLowerLimitDampingUnits=N/(m/s)  PyLowerLimitTransitionRegionWidth=1e-4  PyLowerLimitTransitionRegionWidthUnits=m  PyUpperLimitSpecify=off  PyUpperLimitBound=1  PyUpperLimitBoundUnits=m  PyUpperLimitStiffness=1e6  PyUpperLimitStiffnessUnits=N/m  PyUpperLimitDamping=1e3  PyUpperLimitDampingUnits=N/(m/s)  PyUpperLimitTransitionRegionWidth=1e-4  PyUpperLimitTransitionRegionWidthUnits=m  PyPositionTargetSpecify=on  PyPositionTargetPriority=Low  PyPositionTargetValue=s_b(2,r)  PyPositionTargetValueUnits=m  PyVelocityTargetSpecify=off  PyVelocityTargetPriority=High  PyVelocityTargetValue=0  PyVelocityTargetValueUnits=m/s  PzEquilibriumPosition=0  PzEquilibriumPositionUnits=m  PzSpringStiffness=0  PzSpringStiffnessUnits=N/m  PzDampingCoefficient=0  PzDampingCoefficientUnits=N/(m/s)  PzTorqueActuationMode=NoTorque  PzMotionActuationMode=ComputedMotion  PzSensePosition=on  PzSenseVelocity=on  PzSenseAcceleration=on  PzSenseTorqueForce=off  PzSenseLowerLimitTorqueForce=off  PzSenseUpperLimitTorqueForce=off  PzLowerLimitSpecify=off  PzLowerLimitBound=-1  PzLowerLimitBoundUnits=m  PzLowerLimitStiffness=1e6  PzLowerLimitStiffnessUnits=N/m  PzLowerLimitDamping=1e3  PzLowerLimitDampingUnits=N/(m/s)  PzLowerLimitTransitionRegionWidth=1e-4  PzLowerLimitTransitionRegionWidthUnits=m  PzUpperLimitSpecify=off  PzUpperLimitBound=1  PzUpperLimitBoundUnits=m  PzUpperLimitStiffness=1e6  PzUpperLimitStiffnessUnits=N/m  PzUpperLimitDamping=1e3  PzUpperLimitDampingUnits=N/(m/s)  PzUpperLimitTransitionRegionWidth=1e-4  PzUpperLimitTransitionRegionWidthUnits=m  PzPositionTargetSpecify=on  PzPositionTargetPriority=Low  PzPositionTargetValue=s_b(3,r)  PzPositionTargetValueUnits=m  PzVelocityTargetSpecify=off  PzVelocityTargetPriority=High  PzVelocityTargetValue=0  PzVelocityTargetValueUnits=m/s  RxEquilibriumPosition=0  RxEquilibriumPositionUnits=deg  RxSpringStiffness=0  RxSpringStiffnessUnits=N*m/deg  RxDampingCoefficient=0  RxDampingCoefficientUnits=N*m/(deg/s)  RxTorqueActuationMode=NoTorque  RxMotionActuationMode=ComputedMotion  RxSensePosition=on  RxSenseVelocity=on  RxSenseAcceleration=on  RxSenseTorqueForce=off  RxSenseLowerLimitTorqueForce=off  RxSenseUpperLimitTorqueForce=off  RxLowerLimitSpecify=off  RxLowerLimitBound=-90  RxLowerLimitBoundUnits=deg  RxLowerLimitStiffness=1e4  RxLowerLimitStiffnessUnits=N*m/deg  RxLowerLimitDamping=10  RxLowerLimitDampingUnits=N*m/(deg/s)  RxLowerLimitTransitionRegionWidth=0.1  RxLowerLimitTransitionRegionWidthUnits=deg  RxUpperLimitSpecify=off  RxUpperLimitBound=90  RxUpperLimitBoundUnits=deg  RxUpperLimitStiffness=1e4  RxUpperLimitStiffnessUnits=N*m/deg  RxUpperLimitDamping=10  RxUpperLimitDampingUnits=N*m/(deg/s)  RxUpperLimitTransitionRegionWidth=0.1  RxUpperLimitTransitionRegionWidthUnits=deg  RxPositionTargetSpecify=on  RxPositionTargetPriority=Low  RxPositionTargetValue=s_b(4,r)  RxPositionTargetValueUnits=rad  RxVelocityTargetSpecify=off  RxVelocityTargetPriority=High  RxVelocityTargetValue=0  RxVelocityTargetValueUnits=rad/s  RyEquilibriumPosition=0  RyEquilibriumPositionUnits=deg  RySpringStiffness=0  RySpringStiffnessUnits=N*m/deg  RyDampingCoefficient=0  RyDampingCoefficientUnits=N*m/(deg/s)  RyTorqueActuationMode=NoTorque  RyMotionActuationMode=ComputedMotion  RySensePosition=on  RySenseVelocity=on  RySenseAcceleration=on  RySenseTorqueForce=off  RySenseLowerLimitTorqueForce=off  RySenseUpperLimitTorqueForce=off  RyLowerLimitSpecify=off  RyLowerLimitBound=-90  RyLowerLimitBoundUnits=deg  RyLowerLimitStiffness=1e4  RyLowerLimitStiffnessUnits=N*m/deg  RyLowerLimitDamping=10  RyLowerLimitDampingUnits=N*m/(deg/s)  RyLowerLimitTransitionRegionWidth=0.1  RyLowerLimitTransitionRegionWidthUnits=deg  RyUpperLimitSpecify=off  RyUpperLimitBound=90  RyUpperLimitBoundUnits=deg  RyUpperLimitStiffness=1e4  RyUpperLimitStiffnessUnits=N*m/deg  RyUpperLimitDamping=10  RyUpperLimitDampingUnits=N*m/(deg/s)  RyUpperLimitTransitionRegionWidth=0.1  RyUpperLimitTransitionRegionWidthUnits=deg  RyPositionTargetSpecify=on  RyPositionTargetPriority=Low  RyPositionTargetValue=s_b(5,r)  RyPositionTargetValueUnits=rad  RyVelocityTargetSpecify=off  RyVelocityTargetPriority=High  RyVelocityTargetValue=0  RyVelocityTargetValueUnits=rad/s  RzEquilibriumPosition=0  RzEquilibriumPositionUnits=deg  RzSpringStiffness=0  RzSpringStiffnessUnits=N*m/deg  RzDampingCoefficient=0  RzDampingCoefficientUnits=N*m/(deg/s)  RzTorqueActuationMode=NoTorque  RzMotionActuationMode=ComputedMotion  RzSensePosition=on  RzSenseVelocity=on  RzSenseAcceleration=on  RzSenseTorqueForce=off  RzSenseLowerLimitTorqueForce=off  RzSenseUpperLimitTorqueForce=off  RzLowerLimitSpecify=off  RzLowerLimitBound=-90  RzLowerLimitBoundUnits=deg  RzLowerLimitStiffness=1e4  RzLowerLimitStiffnessUnits=N*m/deg  RzLowerLimitDamping=10  RzLowerLimitDampingUnits=N*m/(deg/s)  RzLowerLimitTransitionRegionWidth=0.1  RzLowerLimitTransitionRegionWidthUnits=deg  RzUpperLimitSpecify=off  RzUpperLimitBound=90  RzUpperLimitBoundUnits=deg  RzUpperLimitStiffness=1e4  RzUpperLimitStiffnessUnits=N*m/deg  RzUpperLimitDamping=10  RzUpperLimitDampingUnits=N*m/(deg/s)  RzUpperLimitTransitionRegionWidth=0.1  RzUpperLimitTransitionRegionWidthUnits=deg  RzPositionTargetSpecify=on  RzPositionTargetPriority=Low  RzPositionTargetValue=s_b(6,r)  RzPositionTargetValueUnits=rad  RzVelocityTargetSpecify=off  RzVelocityTargetPriority=High  RzVelocityTargetValue=0  RzVelocityTargetValueUnits=rad/s
      settings: SourceProductName=Simscape Multibody
  wf : PMIOPort  Side=Left
  G_r : PMIOPort  Port=2  Side=Left
  H_r : PMIOPort  Port=3  Side=Right
  s_r : Outport
  v_r : Outport  Port=2
  a_r : Outport  Port=3
  wires:
  PS-Simulink Converter/1 -> Mux/1
  PS-Simulink Converter3/1 -> Mux/2
  PS-Simulink Converter6/1 -> Mux/3
  PS-Simulink Converter9/1 -> Mux/4
  PS-Simulink Converter12/1 -> Mux/5
  PS-Simulink Converter15/1 -> Mux/6
  Mux/1 -> s_r/1
  PS-Simulink Converter1/1 -> Mux1/1
  PS-Simulink Converter4/1 -> Mux1/2
  PS-Simulink Converter7/1 -> Mux1/3
  PS-Simulink Converter10/1 -> Mux1/4
  PS-Simulink Converter13/1 -> Mux1/5
  PS-Simulink Converter16/1 -> Mux1/6
  Mux1/1 -> v_r/1
  PS-Simulink Converter2/1 -> Mux2/1
  PS-Simulink Converter5/1 -> Mux2/2
  PS-Simulink Converter8/1 -> Mux2/3
  PS-Simulink Converter11/1 -> Mux2/4
  PS-Simulink Converter14/1 -> Mux2/5
  PS-Simulink Converter17/1 -> Mux2/6
  Mux2/1 -> a_r/1
  connections:
  "wf -> O_r"/LConn1 -- wf/RConn1
  body_r/RConn1 -- "O_r -> G_r"/LConn1 -- "wf -> O_r"/RConn1 -- "O_r -> H_r"/LConn1
  H_r/RConn1 -- "O_r -> H_r"/RConn1
  G_r/RConn1 -- "O_r -> G_r"/RConn1
  PS-Simulink Converter/LConn1 -- "wf -> O_r"/RConn2
  "wf -> O_r"/RConn3 -- PS-Simulink Converter1/LConn1
  "wf -> O_r"/RConn4 -- PS-Simulink Converter2/LConn1
  "wf -> O_r"/RConn5 -- PS-Simulink Converter3/LConn1
  "wf -> O_r"/RConn6 -- PS-Simulink Converter4/LConn1
  "wf -> O_r"/RConn7 -- PS-Simulink Converter5/LConn1
  "wf -> O_r"/RConn8 -- PS-Simulink Converter6/LConn1
  "wf -> O_r"/RConn9 -- PS-Simulink Converter7/LConn1
  "wf -> O_r"/RConn10 -- PS-Simulink Converter8/LConn1
  "wf -> O_r"/RConn11 -- PS-Simulink Converter9/LConn1
  "wf -> O_r"/RConn12 -- PS-Simulink Converter10/LConn1
  "wf -> O_r"/RConn13 -- PS-Simulink Converter11/LConn1
  "wf -> O_r"/RConn14 -- PS-Simulink Converter12/LConn1
  "wf -> O_r"/RConn15 -- PS-Simulink Converter13/LConn1
  "wf -> O_r"/RConn16 -- PS-Simulink Converter14/LConn1
  "wf -> O_r"/RConn17 -- PS-Simulink Converter15/LConn1
  "wf -> O_r"/RConn18 -- PS-Simulink Converter16/LConn1
  "wf -> O_r"/RConn19 -- PS-Simulink Converter17/LConn1
